simulink model "MRAC"  (R2018a)
settings: Solver=ode4  StartTime=0.0  StopTime=200  FixedStep=0.1  RelTol=1e-3
undefined symbols (not defined in the file): a, am, b, bm, gamma
settings Model: Creator=klukomski  LastModifiedBy=klukomski

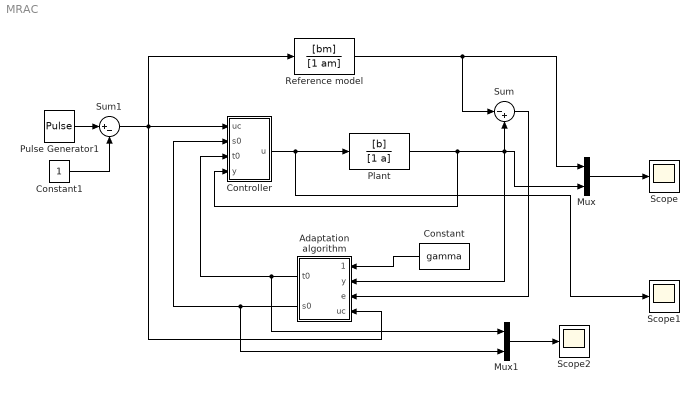
== system MRAC ==
  Adaptation algorithm : Subsystem
  Constant : Constant  Value=gamma
  Constant1 : Constant
  Controller : Subsystem
  Mux : Mux  Inputs=2
  Mux1 : Mux  Inputs=2
  Plant : TransferFcn  Numerator=[b]  Denominator=[1 a]
  Pulse Generator1 : DiscretePulseGenerator  PulseType=Time based  Amplitude=2  Period=20  PulseWidth=50
  Reference model : TransferFcn  Numerator=[bm]  Denominator=[1 am]
  Scope : Scope
  Scope1 : Scope
  Scope2 : Scope
  Sum : Sum  Inputs=|-+
  Sum1 : Sum  Inputs=|+-
  wires:
  Controller/1(u) -> Scope1/1, Plant/1
  Reference model/1 -> Sum/1, Mux/1
  Sum/1 -> Adaptation algorithm/3(e)
  Plant/1 -> Mux/2, Adaptation algorithm/2(y), Sum/2, Controller/4(y)
  Sum1/1 -> Controller/1(uc), Reference model/1, Adaptation algorithm/4(uc)
  Constant/1 -> Adaptation algorithm/1(gamma)
  Mux/1 -> Scope/1
  Pulse Generator1/1 -> Sum1/1
  Constant1/1 -> Sum1/2
  Adaptation algorithm/2(s0) -> Mux1/2, Controller/2(s0)
  Adaptation algorithm/1(t0) -> Mux1/1, Controller/3(t0)
  Mux1/1 -> Scope2/1

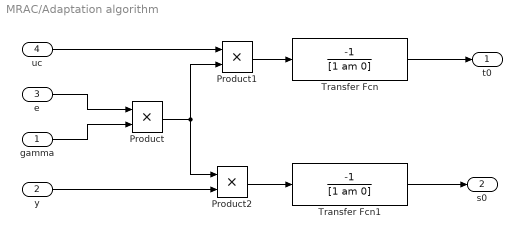
== system MRAC/Adaptation algorithm ==
  gamma : Inport
  y : Inport  Port=2
  e : Inport  Port=3
  uc : Inport  Port=4
  Product : Product
  Product1 : Product
  Product2 : Product
  Transfer Fcn : TransferFcn  Numerator=[-1]  Denominator=[1 am 0]
  Transfer Fcn1 : TransferFcn  Numerator=[-1]  Denominator=[1 am 0]
  t0 : Outport
  s0 : Outport  Port=2
  wires:
  Product/1 -> Product2/1, Product1/2
  Product2/1 -> Transfer Fcn1/1
  uc/1 -> Product1/1
  gamma/1 -> Product/2
  Product1/1 -> Transfer Fcn/1
  y/1 -> Product2/2
  Transfer Fcn1/1 -> s0/1
  Transfer Fcn/1 -> t0/1
  e/1 -> Product/1

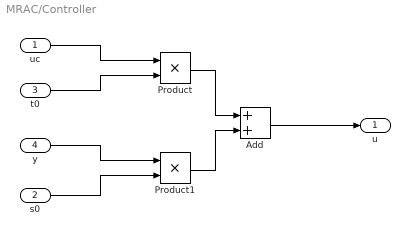
== system MRAC/Controller ==
  uc : Inport
  s0 : Inport  Port=2
  t0 : Inport  Port=3
  y : Inport  Port=4
  Add : Sum
  Product : Product
  Product1 : Product
  u : Outport
  wires:
  Add/1 -> u/1
  Product1/1 -> Add/2
  uc/1 -> Product/1
  Product/1 -> Add/1
  t0/1 -> Product/2
  y/1 -> Product1/1
  s0/1 -> Product1/2
